simulink model "Alcantara_V_MATLAB_No8"  (R2023b)
settings: Solver=VariableStepAuto  StartTime=0.0  StopTime=10.0  RelTol=1e-3
settings Model: Creator=Vincent L. Alcantara  LastModifiedBy=Vincent L. Alcantara

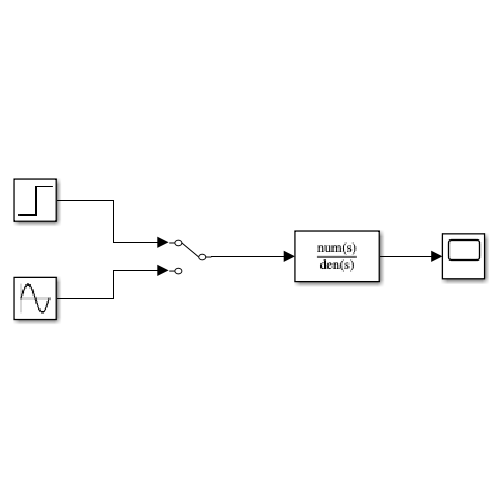
[thumbnail: Simulink's stored preview of the top-level diagram]
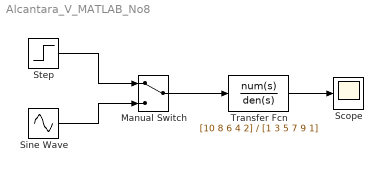
== system Alcantara_V_MATLAB_No8 ==
  Manual Switch : ManualSwitch
  Scope : Scope
  Sine Wave : Sin  SampleTime=0
  Step : Step  Time=0  SampleTime=0
  Transfer Fcn : TransferFcn  Numerator=[10 8 6 4 2]  Denominator=[1 3 5 7 9 1]
  wires:
  Step/1 -> Manual Switch/1
  Sine Wave/1 -> Manual Switch/2
  Manual Switch/1 -> Transfer Fcn/1
  Transfer Fcn/1 -> Scope/1
